simulink model "DCDCconverter"  (R2012b)
settings: Solver=ode3  StartTime=0.0  StopTime=inf  FixedStep=Tsample_simulink  RelTol=1e-3
PostLoadFcn:
  | , if any(exist('dsrtsu_mdlpostloadfcn', 'file') == [2, 3, 6]), try dsrtsu_mdlpostloadfcn('Execute', bdroot); catch fprintf('Error in PostLoadFcn (dsrtsu_mdlpostloadfcn) for model "%s":\n %s\n', bdroot, lasterr); end, end,
InitFcn:
  | load('../sim/me547_based_PI_controller_v3_saved_state.mat');
  | load('../sim/RuleBasedControlData_LeadAcid_48V_25C.mat');
undefined symbols (not defined in the file): BatVoltageLowerThresh, BatVoltageUpperThresh, C, DiscIntNeverNeededParam, Ea, fdesignblkfcn, gcbh, Icommand_Limit, Ireg_Integ_Limit, Kp_vc, MaxBatCurrent, MaxBatVoltage, MaxTemperature, MaxUCCurrent, MaxUCVoltage, Ra, RuleBasedControlHESSPowerValues, RuleBasedControlLUTValues, RuleBasedControlUCVoltageValues, TDelay_UltracapacitorRelay, Ts, Ts2, Tsample_simulink, UCVoltageLowerThresh, UCVoltageUpperThresh, Vbat, Vrail_rated
libraries: xpclib x35, rtilib1103 x8, dspsigops x5
(part 1 of 10)
settings Model: DSRTSU_INTERNAL_RTI_VER=430  DSRTSU_INTERNAL_RTI_TYPE=rti1103  DSRTSU_INTERNAL_RTIFPGA=20  TunableVars=Ea,Ra  TunableVarsStorageClass=Auto,Auto  TunableVarsTypeQualifier=,  BufferReuse=off  Creator=Renato  LastModifiedBy=Raghav
settings DataIOCC: SignalLoggingSaveFormat=ModelDataLogs
settings OptimizationCC: BlockReduction=off  OptimizeBlockIOStorage=off  BufferReuse=off  ExpressionFolding=off  ExpressionDepthLimit=128  LocalBlockOutputs=off
settings DebuggingCC: MultiTaskDSMMsg=warning  MultiTaskCondExecSysMsg=none  StrictBusMsg=None
settings HardwareCC: ProdIntDivRoundTo=Zero  ProdEndianess=BigEndian  ProdHWDeviceType=Generic->Custom  TargetIntDivRoundTo=Zero  TargetEndianess=BigEndian  TargetHWDeviceType=Generic->Custom
settings RTWCC: SystemTargetFile=rti1103.tlc  MakeCommand=make_rti  TemplateMakefile=rti1103.tmf  Description=dSPACE DS1103 Hardware Platform  ProcessScript=rti1103_make_rtw_hook  IncludeERTFirstTime=on
settings STFCustomTargetCC: CodeReplacementLibrary=ANSI_C  ParMdlRefBuildCompliant=on  GeneratePreprocessorConditionals=Disable all  SystemTargetFile=rti1103.tlc
settings GRTTargetCC: CompOptLevelCompliant=off  ConcurrentExecutionCompliant=off  CombineOutputUpdateFcns=off  MatFileLogging=off  GRTInterface=on  ExtModeMexFile=noextcomm

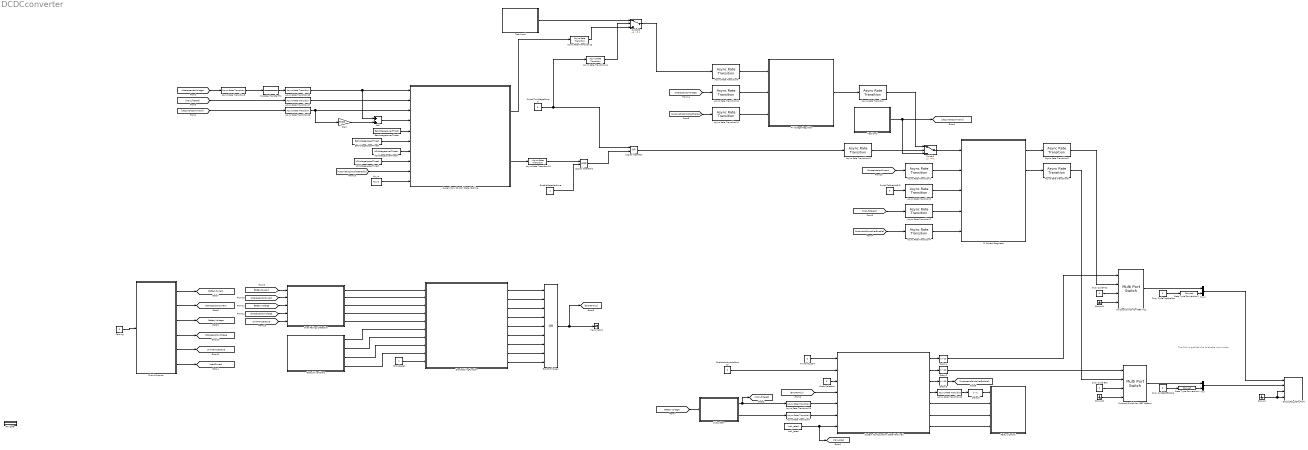
== system DCDCconverter ==
  note: The PWM is enabled whe its enable input is zero
  Add : Sum
  Async Rate Transition{,1..2,4..5,12} (6 alike) : xpclib/Asynchronous Event/Async Rate Transition  sample_time=Ts
  Async Rate Transition{8..11,13..14,16} (7 alike) : xpclib/Asynchronous Event/Async Rate Transition  sample_time=Ts2
  Async Rate Transition15 : xpclib/Asynchronous Event/Async Rate Transition  sample_time=2e-5
  Async Rate Transition17 : xpclib/Asynchronous Event/Async Rate Transition  sample_time=2e-5
  Async Rate Transition18 : xpclib/Asynchronous Event/Async Rate Transition  sample_time=2e-5
  Async Rate Transition19 : xpclib/Asynchronous Event/Async Rate Transition  sample_time=Tsample_simulink
  Async Rate Transition20 : xpclib/Asynchronous Event/Async Rate Transition  sample_time=TDelay_UltracapacitorRelay
  Async Rate Transition3 : xpclib/Asynchronous Event/Async Rate Transition  sample_time=0.00002
  Async Rate Transition6 : xpclib/Asynchronous Event/Async Rate Transition  sample_time=0.00002
  Async Rate Transition7 : xpclib/Asynchronous Event/Async Rate Transition  sample_time=Tsample_simulink
  BatVoltageLowerThresh : Constant  Value=BatVoltageLowerThresh
  BatVoltageUpperThresh : Constant  Value=BatVoltageUpperThresh
  Circuit Outputs : Subsystem
  DS1103SL_DSP_PWM : rtilib1103/DS1103 SLAVE DSP/DS1103SL_DSP_PWM  Parameters=[]  TDef=[]  BoardType=[]  PwmMode=[]  Frequency=[]  InitValue=[]  TermMode=[]  TermValue=[]  Polarity=[]  DialogFcn=[]  Reserved1=[]  Reserved2=[]  Reserved3=[]  Reserved4=[]  Revision=[]  UnitName=[]  UnitValues=[]  DSProperties=struct('RTI',struct('Version',uint32(2),'BlockType',struct('isSLSource',uint8(0),'isSLSink',uint8(1),'isHWSource',uint8(0),'isHWSink',uint8(1),'isSetup',uint8(0),'isInline',uint8(1),'isNonInline',uint8(0),'isInterrupt',uint8(0),'isChannelwise',uint8(0)),'IOBoardType','DS1103SLAVE','UnitType','PWM','Identifier','PWM','DialogType','ML','BlockSet','NONE','SlaveProcessor','F240'))  RTIBlockInterface=struct('InputPortsActive',[1 1 1 1],'InputPortsWidth',int32([2 2 2 2]),'InputPortsName',{{['PWM Channel 1'],['PWM Channel 2'],['PWM Channel 3'],['PWM Channel 4']}},'IWork',{{{'',uint32(4)}}},'DialogFcn','rti1103slavepwmgui','InitLevel',1,'BlockDisplay',{{'','auto'}},'IconTransparency','on','MultiSFcn',4,'BlockName',struct('Token',{{'DS1103SL_DSP_PWM'}}))  RTIBlockParameters=struct('PWMSymmetryMode',{{1,'OFF',[]}},'PWMFrequency',{{'5000','OFF',[]}},'PWMPolarityMode',{{[1 1 1 1 1],'OFF',[]}},'ChannelNo',{{[1 2 3 4],'OFF',[]}},'SuspendModeInit',{{[1 1 1 1 1],'OFF',[]}},'TTLModeInit',{{[2 2 2 2 2],'OFF',[]}},'DutyCycleInitValueCh1',{{'0.5','OFF',[]}},'DutyCycleInitValueCh2',{{'0.5','OFF',[]}},'DutyCycleInitValueCh3',{{'0.5','OFF',[]}},'DutyCycleInitValueCh4',{{'0.5','OFF',[]}},'DutyCycleInitValueCh5',{{'0.5','OFF',[]}},'EnablePWMStop',{{[1 1 1 1 0],'OFF',[]}},'SuspendModeTerm',{{[1 1 1 1 1],'OFF',[]}},'TTLModeTerm',{{[2 2 2 2 2],'OFF',[]}},'DutyCycleTermValueCh1',{{'0.5','OFF',[]}},'DutyCycleTermValueCh2',{{'0.5','OFF',[]}},'DutyCycleTermValueCh3',{{'0.5','OFF',[]}},'DutyCycleTermValueCh4',{{'0.5','OFF',[]}},'DutyCycleTermValueCh5',{{'0.5','OFF',[]}},'TLCFileName',{{'rti1103pwm','OFF',[]}})  RTISFcnParameters=struct('PWMSymmetryMode','double','PWMFrequency','double','PWMPolarityMode','double','ChannelNo','double','SuspendModeInit','double','TTLModeInit','double','DutyCycleInitValueCh1','double','DutyCycleInitValueCh2','double','DutyCycleInitValueCh3','double','DutyCycleInitValueCh4','double','EnablePWMStop','double','SuspendModeTerm','double','TTLModeTerm','double','DutyCycleTermValueCh1','double','DutyCycleTermValueCh2','double','DutyCycleTermValueCh3','double','DutyCycleTermValueCh4','double','TLCFileName','char')  RTIBlockParaDefault=struct('PWMSymmetryMode',1,'PWMFrequency',100,'PWMPolarityMode',[1 1 1 1 1],'ChannelNo',[1 2 3 4],'SuspendModeInit',[1 1 1 1 1],'TTLModeInit',[2 2 2 2 2],'DutyCycleInitValueCh1',0.5,'DutyCycleInitValueCh2',0.5,'DutyCycleInitValueCh3',0.5,'DutyCycleInitValueCh4',0.5,'DutyCycleInitValueCh5',0.5,'EnablePWMStop',[1 1 1 1 0],'SuspendModeTerm',[1 1 1 1 1],'TTLModeTerm',[2 2 2 2 2],'DutyCycleTermValueCh1',0.5,'DutyCycleTermValueCh2',0.5,'DutyCycleTermValueCh3',0.5,'DutyCycleTermValueCh4',0.5,'DutyCycleTermValueCh5',0.5,'TLCFileName','rti1103pwm')
  Data Type Conversion1 : DataTypeConversion
  Data Type Conversion2 : DataTypeConversion
  Delay1 : Delay  DelayLength=10  SampleTime=Tsample_simulink
  Delay2 : Delay  DelayLength=10  SampleTime=Tsample_simulink
  Delay3 : Delay  DelayLength=10  SampleTime=Tsample_simulink
  Delay5 : Delay  DelayLength=1  SampleTime=TDelay_UltracapacitorRelay
  Discrete Transfer Fcn : DiscreteTransferFcn  Numerator=[1 1 1 1]  Denominator=[4 0 0 0]  SampleTime=Ts2
  Duty Cycle Bot : Constant  Value=0
  Duty CycleBotEnable : Constant  Value=0
  Duty CycleTop : Constant  Value=0
  Duty CycleTopEnable : Constant  Value=0
  EnableAutomaticControl : Constant  Value=0
  EnableStateMachine : Constant  SampleTime=-1
  ErrorForTripNew : Logic  Operator=OR  Inputs=9  AllPortsSameDT=off  OutDataTypeStr=boolean
  ErrorLatchingFunction : MATLAB Function  TreatAsAtomicUnit=on
  Error_Reset : Constant
  Gain : Gain  Gain=Ts2/C
  Gate Driver Errors : Subsystem
  Ground : Ground
  Ground1 : Ground
  Ground2 : Ground
  Kp_vc : Constant  Value=Kp_vc  SampleTime=-1
  Logical Operator : Logic  Operator=OR  AllPortsSameDT=off  OutDataTypeStr=boolean
  Logical Operator1 : Logic  AllPortsSameDT=off  OutDataTypeStr=boolean
  Mode Selection : Constant  Value=0
  Multiport Switch for IGBT Bottom : MultiPortSwitch  Inputs=2  DataPortForDefault=Additional data port  DiagnosticForDefault=None
  Multiport Switch for IGBT Top : MultiPortSwitch  Inputs=2  DataPortForDefault=Additional data port  DiagnosticForDefault=None
  Mux : Mux  Inputs=2
  Mux1 : Mux  Inputs=2
  Over Ratings Detection : Subsystem
  PI Current Regulator : Subsystem
  PI Voltage Regulator : Subsystem
  RTI Data : Subsystem  Tag=struct('RTIDataServer',struct('RTIDataServerVs','2','RTIModelDescription','struct(''main'',''DCDCconverter'',''sub'','''',''isMp'',0)'))  LoadFcn="if exist('rtidc'), try,  rtidc('DataHostBlockClbLoad', gcbh); catch, disp(['Warning: ''LoadFcn'' for RTI Data block failed: ' lasterr]); end, end,"  mask(RTI_DATA_HOST){}
      mask help:
      | RTI Data Block.
      | This block is used by RTI to store internal model-dependent data.
      | Please keep this block on the root level of the model. Deleting this block will result in data loss.
      |
      | NEVER DELETE OR COPY THIS BLOCK!
      settings: CopyFcn="if exist('rtidc'), try,  rtidc('DataHostBlockClbCopy', gcbh); catch, disp(['Warning: ''CopyFcn'' for RTI Data block failed: ' lasterr]); end, end,"  DeleteFcn="if exist('rtidc'), try,  rtidc('DataHostBlockClbDelete', gcbh); catch, disp(['Warning: ''DeleteFcn'' for RTI Data block failed: ' lasterr]); end, end,"  ModelCloseFcn="if exist('rtidc'), try,  rtidc('DataHostBlockClbModelClose', gcbh); catch, disp(['Warning: ''ModelCloseFcn'' for RTI Data block failed: ' lasterr]); end, end,"  PreSaveFcn="if exist('rtidc'), try,  rtidc('DataHostBlockClbPreSave', gcbh); catch, disp(['Warning: ''PreSaveFcn'' for RTI Data block failed: ' lasterr]); end, end,"  PostSaveFcn="if exist('rtidc'), try,  rtidc('DataHostBlockClbPostSave', gcbh); catch, disp(['Warning: ''PostSaveFcn'' for RTI Data block failed: ' lasterr]); end, end,"  NameChangeFcn="if exist('rtidc'), try,  rtidc('DataHostBlockClbNameChange', gcbh); catch, disp(['Warning: ''NameChangeFcn'' for RTI Data block failed: ' lasterr]); end, end,"
      mask Help:
      | RTI Data Block.
      | This block is used by RTI to store internal model-dependent data.
      | Please keep this block on the root level of the model. Deleting this block will result in data loss.
      | 
      | NEVER DELETE OR COPY THIS BLOCK!
      mask Display:
      | text(0.5, 0.5, 'RTI Data', 'HorizontalAlignment', 'center');
      | plot([1 0]);
  Relays Control : Subsystem
  Subsystem : Subsystem
  Supervisory Control State Machine : Stateflow chart  TreatAsAtomicUnit=on
  Switch2 : Switch  Threshold=1  OutDataTypeStr=Inherit: Inherit via back propagation  SampleTime=Ts
  Switch5 : Switch  Threshold=1  OutDataTypeStr=Inherit: Inherit via back propagation  SampleTime=Ts2
  SwitchToEnableDID : Constant  Value=0
  SwitchToVoltageControl : Constant  Value=0  SampleTime=-1
  System Configuration State Machine1 : Stateflow chart  TreatAsAtomicUnit=on
  Terminator1 : Terminator
  Test Icmd : Subsystem
  Test Vcmd : Subsystem
  TurnOnSystem : Constant  Value=0
  UCVoltageLowerThresh : Constant  Value=UCVoltageLowerThresh
  UCVoltageUpperThresh : Constant  Value=UCVoltageUpperThresh
  Vrail_rated : Constant  Value=Vrail_rated
  Zeroing : Constant  Value=0
  tag scope: BatteryCurrent=global, BatteryVoltage=global, LoadCurrent=global, SinkTemperature=global, UltracapacitorCurrent=global, UltracapacitorVoltage=global, Vrail_rated=global
  wires:
  Data Type Conversion1/1 -> Mux/2
  Over Ratings Detection/5(Temperature Alert) -> ErrorLatchingFunction/5(TempAlert)
  Over Ratings Detection/4(Ultracapacitor Voltage Alert) -> ErrorLatchingFunction/4(UCVoltageAlert)
  Over Ratings Detection/3(Battery Voltage Alert) -> ErrorLatchingFunction/3(BatVoltageAlert)
  Over Ratings Detection/2(Ultra Capacitor Current Alert) -> ErrorLatchingFunction/2(UCCurrentAlert)
  Over Ratings Detection/1(Battery Current Alert) -> ErrorLatchingFunction/1(BatCurrentAlert)
  Mux/1 -> DS1103SL_DSP_PWM/2
  Gate Driver Errors/1(Error HB1) -> ErrorLatchingFunction/6(ErrorHB1)
  Gate Driver Errors/2(Error HB2) -> ErrorLatchingFunction/7(ErrorHB2)
  Gate Driver Errors/3(Error HB3) -> ErrorLatchingFunction/8(ErrorHB3)
  Gate Driver Errors/4(Over Temperature) -> ErrorLatchingFunction/9(OverTemp)
  Duty CycleTop/1 -> Multiport Switch for IGBT Top/3
  Data Type Conversion2/1 -> Mux1/2
  Mux1/1 -> DS1103SL_DSP_PWM/1
  Ground/1 -> DS1103SL_DSP_PWM/3, DS1103SL_DSP_PWM/4
  Zeroing/1 -> Circuit Outputs/1(Zeroing)
  Multiport Switch for IGBT Top/1 -> Mux1/1
  Multiport Switch for IGBT Bottom/1 -> Mux/1
  PI Current Regulator/1(Duty Cycle Command Top) -> Async Rate Transition3/1
  Duty Cycle Bot/1 -> Multiport Switch for IGBT Bottom/3
  EnableAutomaticControl/1 -> System Configuration State Machine1/2(EnableAutomaticControl)
  Async Rate Transition1/1 -> PI Current Regulator/2(Avg Current Measurement)
  Async Rate Transition2/1 -> PI Current Regulator/4(DC Bus Voltage Measurement)
  SwitchToEnableDID/1 -> Async Rate Transition5/1
  Async Rate Transition4/1 -> PI Current Regulator/5(Enable PI Controller)
  Async Rate Transition5/1 -> PI Current Regulator/3(Enable DID)
  PI Current Regulator/2(Duty Cycle Command Bottom) -> Async Rate Transition6/1
  Duty CycleTopEnable/1 -> Data Type Conversion2/1
  Duty CycleBotEnable/1 -> Data Type Conversion1/1
  Async Rate Transition3/1 -> Multiport Switch for IGBT Top/2
  Async Rate Transition6/1 -> Multiport Switch for IGBT Bottom/2
  Async Rate Transition9/1 -> PI Voltage Regulator/1(UC Voltage Command)
  Async Rate Transition10/1 -> PI Voltage Regulator/2(UC Voltage Measurement)
  Async Rate Transition11/1 -> PI Voltage Regulator/3(Enable PI Controller)
  Test Icmd/1(Current Command) -> [UCCurrentCommand], Switch2/3
  PI Voltage Regulator/1(Avg Current Command) -> Async Rate Transition/1
  Switch2/1 -> PI Current Regulator/1(Avg Current Command)
  Async Rate Transition/1 -> Switch2/1
  BatVoltageLowerThresh/1 -> Supervisory Control State Machine/5(BatVoltageLowerThresh)
  BatVoltageUpperThresh/1 -> Supervisory Control State Machine/6(BatVoltageUpperThresh)
  UCVoltageLowerThresh/1 -> Supervisory Control State Machine/7(UCVoltageLowerThresh)
  UCVoltageUpperThresh/1 -> Supervisory Control State Machine/8(UCVoltageUpperThresh)
  Supervisory Control State Machine/2(EnableVoltageCommand) -> Async Rate Transition16/1
  EnableStateMachine/1 -> Logical Operator1/2
  Test Vcmd/1(Voltage Command) -> Switch5/1
  Switch5/1 -> Async Rate Transition9/1
  [UltracapacitorVoltage] -> Async Rate Transition8/1
  Gain/1 -> Add/2
  Logical Operator/1 -> Async Rate Transition12/1
  Logical Operator1/1 -> Logical Operator/2
  Async Rate Transition12/1 -> Switch2/2
  Supervisory Control State Machine/1(VoltageCommand) -> Async Rate Transition13/1
  SwitchToVoltageControl/1 -> Async Rate Transition14/1, Logical Operator/1
  Discrete Transfer Fcn/1 -> Async Rate Transition15/1
  [Vrail_filtered] -> Async Rate Transition17/1
  [UCCurrentCommand] -> Async Rate Transition18/1
  Async Rate Transition13/1 -> Switch5/3
  Async Rate Transition14/1 -> Switch5/2
  Async Rate Transition15/1 -> Supervisory Control State Machine/1(Average_UCVoltage), Add/1
  Async Rate Transition17/1 -> Supervisory Control State Machine/2(Average_BatVoltage)
  Async Rate Transition18/1 -> Supervisory Control State Machine/3(UCCurrentCommand), Gain/1
  Add/1 -> Supervisory Control State Machine/4(UCVoltage_next_predicted)
  Ground1/1 -> Multiport Switch for IGBT Top/4
  Ground2/1 -> Multiport Switch for IGBT Bottom/4
  Delay2/1 -> Multiport Switch for IGBT Bottom/1
  Subsystem/1(Vrail_filtered) -> Async Rate Transition19/1, [Vrail_filtered]
  Subsystem/2(dVrail_dT_filtered) -> Async Rate Transition7/1
  [Vrail_filtered] -> Async Rate Transition2/1
  Async Rate Transition19/1 -> System Configuration State Machine1/5(Vrail)
  Async Rate Transition7/1 -> System Configuration State Machine1/6(dVrail_dT)
  Vrail_rated/1 -> [Vrail_rated], System Configuration State Machine1/7(Vrail_rated)
  [ErrorForTrip] -> System Configuration State Machine1/4(Error)
  Mode Selection/1 -> System Configuration State Machine1/3(ManualControlBuckMode)
  System Configuration State Machine1/4(UltracapacitorRelay) -> Async Rate Transition20/1
  System Configuration State Machine1/5(ChargingRelay) -> Relays Control/2(Charging Relay)
  System Configuration State Machine1/6(DischargingRelay) -> Relays Control/3(Discharging Relay)
  System Configuration State Machine1/7(BatteryRelay) -> Relays Control/4(Battery Relay)
  Delay3/1 -> [AutomaticControllerEnable]
  Circuit Outputs/1(Battery Current) -> [BatteryCurrent]
  Circuit Outputs/2(UltraCapacitor Current) -> [UltracapacitorCurrent]
  Circuit Outputs/3(Battery Voltage) -> [BatteryVoltage]
  Circuit Outputs/4(UltraCapacitor Voltage) -> [UltracapacitorVoltage]
  Circuit Outputs/5(Sink Temperature) -> [SinkTemperature]
  [BatteryVoltage] -> Subsystem/1(Vrail)
  TurnOnSystem/1 -> System Configuration State Machine1/1(TurnOnSystem)
  [AutomaticControllerEnable] -> Async Rate Transition4/1
  [AutomaticControllerEnable] -> Async Rate Transition11/1
  Delay1/1 -> Multiport Switch for IGBT Top/1
  System Configuration State Machine1/2(IGBT_Bot_State) -> Delay2/1
  System Configuration State Machine1/3(AutomaticController) -> Delay3/1
  System Configuration State Machine1/1(IGBT_Top_State) -> Delay1/1
  [BatteryCurrent] -> Over Ratings Detection/1(Battery Current)
  [UltracapacitorCurrent] -> Over Ratings Detection/2(Ultra Capacitor Current)
  [BatteryVoltage] -> Over Ratings Detection/3(Battery Voltage)
  [UltracapacitorVoltage] -> Over Ratings Detection/4(Ultra Capacitor Voltage)
  [SinkTemperature] -> Over Ratings Detection/5(Temperature)
  [UltracapacitorVoltage] -> Async Rate Transition10/1
  [UltracapacitorCurrent] -> Async Rate Transition1/1
  [AutomaticControllerEnable] -> Supervisory Control State Machine/9(AutomaticControllerEnable)
  Kp_vc/1 -> Supervisory Control State Machine/10(Kp_vc)
  ErrorLatchingFunction/3(LBatVoltageAlert) -> ErrorForTripNew/3
  ErrorLatchingFunction/2(LUCCurrentAlert) -> ErrorForTripNew/2
  ErrorLatchingFunction/4(LUCVoltageAlert) -> ErrorForTripNew/4
  ErrorLatchingFunction/7(LErrorHB2) -> ErrorForTripNew/7
  ErrorLatchingFunction/5(LTempAlert) -> ErrorForTripNew/5
  ErrorLatchingFunction/8(LErrorHB3) -> ErrorForTripNew/8
  ErrorLatchingFunction/6(LErrorHB1) -> ErrorForTripNew/6
  ErrorLatchingFunction/9(LOverTemp) -> ErrorForTripNew/9
  ErrorLatchingFunction/1(LBatCurrentAlert) -> ErrorForTripNew/1
  ErrorForTripNew/1 -> [ErrorForTrip], Terminator1/1
  Error_Reset/1 -> ErrorLatchingFunction/10(Error_Reset)
  Async Rate Transition8/1 -> Discrete Transfer Fcn/1
  Circuit Outputs/6(Load Current) -> [LoadCurrent]
  Async Rate Transition16/1 -> Logical Operator1/1
  Delay5/1 -> Relays Control/1(UltraCapacitor Relay)
  Async Rate Transition20/1 -> Delay5/1

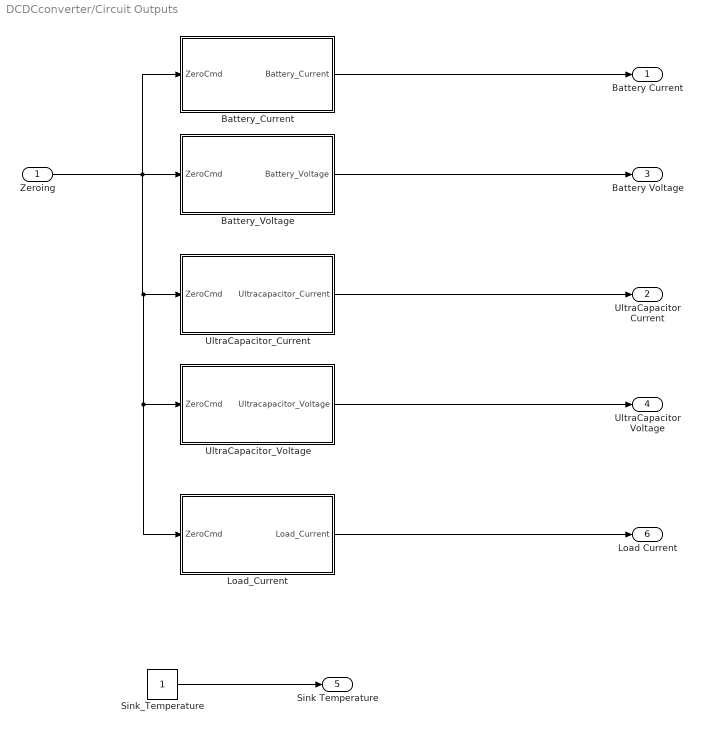
== system DCDCconverter/Circuit Outputs ==
  Zeroing : Inport
  Battery_Current : Subsystem
  Battery_Voltage : Subsystem
  Load_Current : Subsystem
  Sink_Temperature : Constant
  UltraCapacitor_Current : Subsystem
  UltraCapacitor_Voltage : Subsystem
  Battery Current : Outport
  UltraCapacitor Current : Outport  Port=2
  Battery Voltage : Outport  Port=3
  UltraCapacitor Voltage : Outport  Port=4
  Sink Temperature : Outport  Port=5
  Load Current : Outport  Port=6
  wires:
  Battery_Voltage/1(Battery_Voltage) -> Battery Voltage/1
  Battery_Current/1(Battery_Current) -> Battery Current/1
  Sink_Temperature/1 -> Sink Temperature/1
  Zeroing/1 -> Load_Current/1(ZeroCmd), UltraCapacitor_Voltage/1(ZeroCmd), UltraCapacitor_Current/1(ZeroCmd), Battery_Voltage/1(ZeroCmd), Battery_Current/1(ZeroCmd)
  UltraCapacitor_Voltage/1(Ultracapacitor_Voltage) -> UltraCapacitor Voltage/1
  UltraCapacitor_Current/1(Ultracapacitor_Current) -> UltraCapacitor Current/1
  Load_Current/1(Load_Current) -> Load Current/1

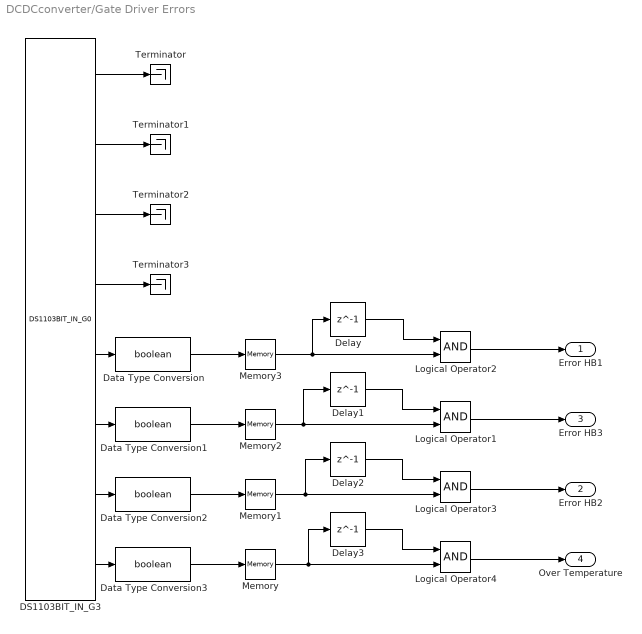
== system DCDCconverter/Gate Driver Errors ==
  DS1103BIT_IN_G3 : rtilib1103/DS1103 MASTER PPC/DS1103BIT_IN_G0  GroupNo=3  Reserved1=[]  Reserved2=[]  Reserved3=[]  Reserved4=[]  DialogFcn=gui1103bit_inx  UnitName={ 'DS1103BIT_IN_G'}  UnitValues={ 3 }  DSProperties=struct('RTI',struct('Version',uint32(1),'BlockType',struct('isSLSource',uint8(1),'isSLSink',uint8(0),'isHWSource',uint8(1),'isHWSink',uint8(0),'isSetup',uint8(0),'isInline',uint8(1),'isNonInline',uint8(0),'isInterrupt',uint8(0),'isChannelwise',uint8(0)),'IOBoardType','DS1103MASTER','UnitType','BIT','Identifier','BITIN','DialogType','ML','BlockSet','NONE','SlaveProcessor','NONE'))
  Data Type Conversion{,1..3} (4 alike) : DataTypeConversion  OutDataTypeStr=boolean
  Delay{,1..3} (4 alike) : Delay  DelayLength=1
  Logical Operator{1..4} (4 alike) : Logic  AllPortsSameDT=off  OutDataTypeStr=boolean
  Memory{,1..3} (4 alike) : Memory  InheritSampleTime=on
  Terminator{,1..3} (4 alike) : Terminator
  Error HB1 : Outport
  Error HB2 : Outport  Port=2
  Error HB3 : Outport  Port=3
  Over Temperature : Outport  Port=4
  wires:
  DS1103BIT_IN_G3/1 -> Terminator/1
  DS1103BIT_IN_G3/4 -> Terminator3/1
  DS1103BIT_IN_G3/2 -> Terminator1/1
  DS1103BIT_IN_G3/3 -> Terminator2/1
  DS1103BIT_IN_G3/8 -> Data Type Conversion3/1
  DS1103BIT_IN_G3/6 -> Data Type Conversion1/1
  DS1103BIT_IN_G3/7 -> Data Type Conversion2/1
  DS1103BIT_IN_G3/5 -> Data Type Conversion/1
  Data Type Conversion3/1 -> Memory/1
  Data Type Conversion2/1 -> Memory1/1
  Data Type Conversion1/1 -> Memory2/1
  Data Type Conversion/1 -> Memory3/1
  Memory3/1 -> Delay/1, Logical Operator2/2
  Logical Operator2/1 -> Error HB1/1
  Delay/1 -> Logical Operator2/1
  Memory2/1 -> Delay1/1, Logical Operator1/2
  Logical Operator1/1 -> Error HB3/1
  Delay1/1 -> Logical Operator1/1
  Logical Operator3/1 -> Error HB2/1
  Memory1/1 -> Delay2/1, Logical Operator3/2
  Delay2/1 -> Logical Operator3/1
  Logical Operator4/1 -> Over Temperature/1
  Memory/1 -> Logical Operator4/2, Delay3/1
  Delay3/1 -> Logical Operator4/1

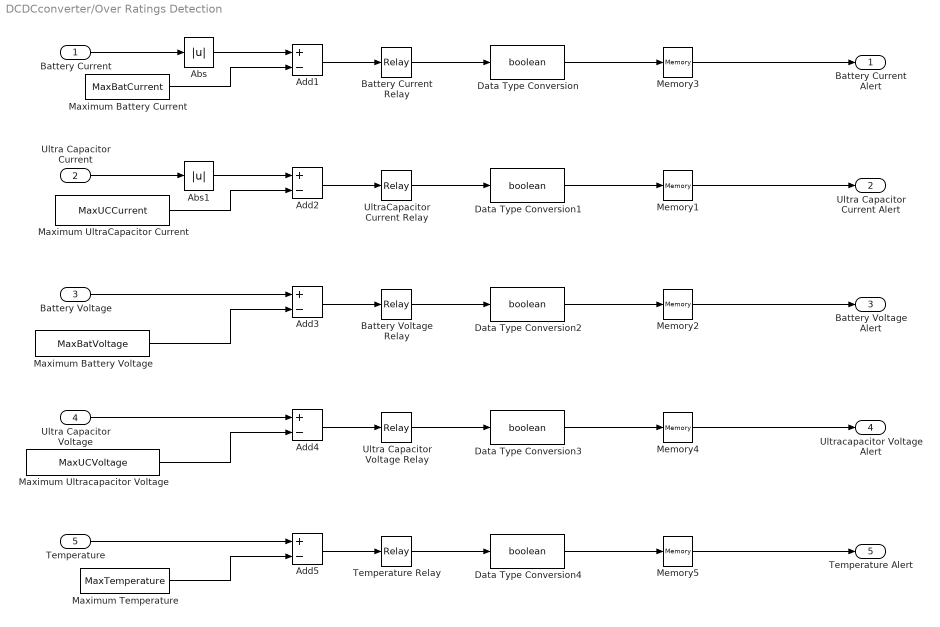
== system DCDCconverter/Over Ratings Detection ==
  Battery Current : Inport
  Ultra Capacitor Current : Inport  Port=2
  Battery Voltage : Inport  Port=3
  Ultra Capacitor Voltage : Inport  Port=4
  Temperature : Inport  Port=5
  Abs : Abs
  Abs1 : Abs
  Add{1..5} (5 alike) : Sum  Inputs=+-
  Battery Current Relay : Relay  OnSwitchValue=0  OffSwitchValue=0
  Battery Voltage Relay : Relay  OnSwitchValue=0  OffSwitchValue=0
  Data Type Conversion{,1..4} (5 alike) : DataTypeConversion  OutDataTypeStr=boolean
  Maximum Battery Current : Constant  Value=MaxBatCurrent
  Maximum Battery Voltage : Constant  Value=MaxBatVoltage
  Maximum Temperature : Constant  Value=MaxTemperature
  Maximum UltraCapacitor Current : Constant  Value=MaxUCCurrent
  Maximum Ultracapacitor Voltage : Constant  Value=MaxUCVoltage
  Memory{1..5} (5 alike) : Memory  InheritSampleTime=on
  Temperature Relay : Relay  OnSwitchValue=0  OffSwitchValue=0
  Ultra Capacitor Voltage Relay : Relay  OnSwitchValue=0  OffSwitchValue=0
  UltraCapacitor Current Relay : Relay  OnSwitchValue=0  OffSwitchValue=0
  Battery Current Alert : Outport
  Ultra Capacitor Current Alert : Outport  Port=2
  Battery Voltage Alert : Outport  Port=3
  Ultracapacitor Voltage Alert : Outport  Port=4
  Temperature Alert : Outport  Port=5
  wires:
  Add3/1 -> Battery Voltage Relay/1
  Maximum Battery Voltage/1 -> Add3/2
  Battery Voltage/1 -> Add3/1
  Add4/1 -> Ultra Capacitor Voltage Relay/1
  Maximum Ultracapacitor Voltage/1 -> Add4/2
  Ultra Capacitor Voltage/1 -> Add4/1
  Add2/1 -> UltraCapacitor Current Relay/1
  Maximum UltraCapacitor Current/1 -> Add2/2
  Ultra Capacitor Current/1 -> Abs1/1
  Add5/1 -> Temperature Relay/1
  Maximum Temperature/1 -> Add5/2
  Temperature/1 -> Add5/1
  Add1/1 -> Battery Current Relay/1
  Maximum Battery Current/1 -> Add1/2
  Battery Current/1 -> Abs/1
  Battery Current Relay/1 -> Data Type Conversion/1
  UltraCapacitor Current Relay/1 -> Data Type Conversion1/1
  Battery Voltage Relay/1 -> Data Type Conversion2/1
  Ultra Capacitor Voltage Relay/1 -> Data Type Conversion3/1
  Temperature Relay/1 -> Data Type Conversion4/1
  Data Type Conversion/1 -> Memory3/1
  Data Type Conversion1/1 -> Memory1/1
  Data Type Conversion2/1 -> Memory2/1
  Data Type Conversion3/1 -> Memory4/1
  Data Type Conversion4/1 -> Memory5/1
  Memory3/1 -> Battery Current Alert/1
  Memory1/1 -> Ultra Capacitor Current Alert/1
  Memory2/1 -> Battery Voltage Alert/1
  Memory4/1 -> Ultracapacitor Voltage Alert/1
  Memory5/1 -> Temperature Alert/1
  Abs/1 -> Add1/1
  Abs1/1 -> Add2/1

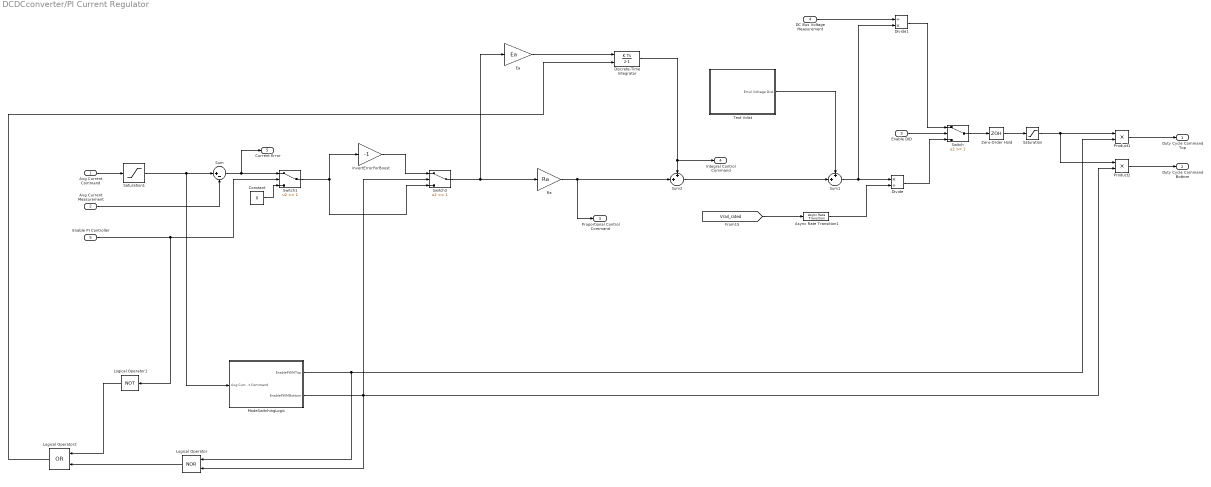
== system DCDCconverter/PI Current Regulator ==
  Avg Current Command : Inport
  Avg Current Measurement : Inport  Port=2
  Enable DID : Inport  Port=3
  DC Bus Voltage Measurement : Inport  Port=4
  Enable PI Controller : Inport  Port=5
  Async Rate Transition1 : xpclib/Asynchronous Event/Async Rate Transition  sample_time=Ts
  Constant : Constant  Value=0  SampleTime=Ts
  Discrete-Time Integrator : DiscreteIntegrator  ExternalReset=either  SampleTime=Ts  LimitOutput=on  UpperSaturationLimit=Ireg_Integ_Limit  LowerSaturationLimit=-Ireg_Integ_Limit  ICPrevOutput=DiscIntNeverNeededParam  ICPrevScaledInput=DiscIntNeverNeededParam
  Divide : Product  Inputs=*/
  Divide1 : Product  Inputs=/*
  Ea : Gain  Gain=Ea  SampleTime=Ts
  InvertErrorForBoost : Gain  Gain=-1  SampleTime=Ts
  Logical Operator : Logic  Operator=NOR  AllPortsSameDT=off  OutDataTypeStr=boolean
  Logical Operator1 : Logic  Operator=NOT  AllPortsSameDT=off  OutDataTypeStr=boolean
  Logical Operator2 : Logic  Operator=OR  AllPortsSameDT=off  OutDataTypeStr=boolean
  ModeSwitchingLogic : Subsystem
  Product1 : Product  RndMeth=Zero
  Product2 : Product  RndMeth=Zero
  Ra : Gain  Gain=Ra  SampleTime=Ts
  Saturation : Saturate  UpperLimit=1  LowerLimit=0
  Saturation1 : Saturate  UpperLimit=Icommand_Limit  LowerLimit=-Icommand_Limit
  Sum : Sum  Inputs=|+-
  Sum1 : Sum  Inputs=++|
  Sum2 : Sum  Inputs=++|
  Switch : Switch  Threshold=1
  Switch1 : Switch  Threshold=1
  Switch3 : Switch  Threshold=1
  Test Vdist : Subsystem
  Zero-Order Hold : ZeroOrderHold  SampleTime=Ts
  Duty Cycle Command Top : Outport
  Duty Cycle Command Bottom : Outport  Port=2
  Proportional Control Command : Outport  Port=3
  Integral Control Command : Outport  Port=4
  Current Error : Outport  Port=5
  wires:
  Divide/1 -> Switch/3
  Ea/1 -> Discrete-Time Integrator/1
  Zero-Order Hold/1 -> Saturation/1
  Ra/1 -> Proportional Control Command/1, Sum2/2
  Discrete-Time Integrator/1 -> Sum2/1, Integral Control Command/1
  Switch/1 -> Zero-Order Hold/1
  Enable DID/1 -> Switch/2
  DC Bus Voltage Measurement/1 -> Divide1/1
  Divide1/1 -> Switch/1
  Sum/1 -> Current Error/1, Switch1/1
  Constant/1 -> Switch1/3
  Avg Current Command/1 -> Saturation1/1
  Avg Current Measurement/1 -> Sum/2
  Enable PI Controller/1 -> Logical Operator1/1, Switch1/2
  Saturation/1 -> Product2/1, Product1/1
  ModeSwitchingLogic/1(EnablePWMTop) -> Product1/2, Logical Operator/1
  ModeSwitchingLogic/2(EnablePWMBottom) -> Logical Operator/2, Product2/2, Switch3/2
  Sum2/1 -> Sum1/2
  Sum1/1 -> Divide1/2, Divide/1
  Test Vdist/1(Emul Voltage Dist) -> Sum1/1
  Logical Operator2/1 -> Discrete-Time Integrator/2
  Switch1/1 -> Switch3/3, InvertErrorForBoost/1
  InvertErrorForBoost/1 -> Switch3/1
  Switch3/1 -> Ea/1, Ra/1
  Saturation1/1 -> ModeSwitchingLogic/1(Avg Current Command), Sum/1
  Logical Operator1/1 -> Logical Operator2/1
  Logical Operator/1 -> Logical Operator2/2
  Product1/1 -> Duty Cycle Command Top/1
  Product2/1 -> Duty Cycle Command Bottom/1
  [Vrail_rated] -> Async Rate Transition1/1
  Async Rate Transition1/1 -> Divide/2

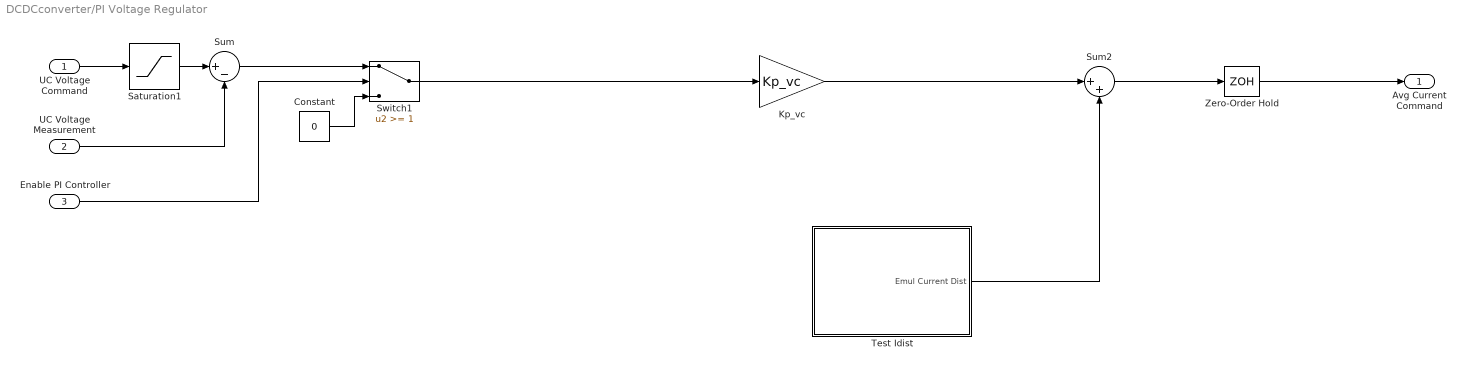
== system DCDCconverter/PI Voltage Regulator ==
  UC Voltage Command : Inport
  UC Voltage Measurement : Inport  Port=2
  Enable PI Controller : Inport  Port=3
  Constant : Constant  Value=0  SampleTime=Ts2
  Kp_vc : Gain  Gain=Kp_vc  SampleTime=Ts2
  Saturation1 : Saturate  UpperLimit=Vbat-1  LowerLimit=0
  Sum : Sum  Inputs=|+-
  Sum2 : Sum  Inputs=|++
  Switch1 : Switch  Threshold=1
  Test Idist : Subsystem
  Zero-Order Hold : ZeroOrderHold  SampleTime=Ts2
  Avg Current Command : Outport
  wires:
  Switch1/1 -> Kp_vc/1
  Sum/1 -> Switch1/1
  Constant/1 -> Switch1/3
  UC Voltage Command/1 -> Saturation1/1
  UC Voltage Measurement/1 -> Sum/2
  Enable PI Controller/1 -> Switch1/2
  Zero-Order Hold/1 -> Avg Current Command/1
  Saturation1/1 -> Sum/1
  Sum2/1 -> Zero-Order Hold/1
  Kp_vc/1 -> Sum2/1
  Test Idist/1(Emul Current Dist) -> Sum2/2

== system DCDCconverter/RTI Data ==
  RTI Data Store : Subsystem  Tag="struct('public',struct('sub',struct('name',{{'DCDCconverter'}},'data',{{struct('TH',struct('thTaskInfo',struct('taskType',{'TIMER','HWINT','TMRINT','SWINT','GLINT'},'tasksNumOf',{4,0,0,0,0},'srcIds',{{'TIMERA','TIMERA2','TIMERA3','TIMERA4'},{},{},{},{}},'taskNames',{{['Timer Task 1'],['Timer Task 2'],['Timer Task 3'],['Timer Task 4']},{},{},{},{}})),'th_tc',struct('dataType',{'TASK','TASK','TASK','TASK'},'taskGroupId',{'','','',''},'taskGroupList',{{},{},{},{}},'taskSchedulingPolicy',{'FCFS','FCFS','FCFS','FCFS'},'taskType',{'TIMER','TIMER','TIMER','TIMER'},'blkh',{-1,-1,-1,-1},'srcId',{'TIMERA','TIMERA2','TIMERA3','TIMERA4'},'srcSgnName',{['Timer A interrupt'],['Timer Task 1'],['Timer Task 1'],['Timer Task 1']},'srcCpuName',{'','','',''},'taskName',{['Timer Task 1  [2e-05] s'],['Timer Task 2  [0.0002] s'],['Timer Task 3  [0.05] s'],['Timer Task 4  [0.5] s']},'taskNameDisplayExt',{'','','',''},'smplTime',{2e-05,0.0002,0.05,0.5},'smplTimeOffs',{0,0,0,0},'hasFixedPriority',{0,0,0,0},'priority',{1,2,3,4},'hasFixedOvc',{0,0,0,0},'ovcType',{1,1,1,1},'ovcMax',{1,1,1,1}),'tc_th',struct('dataType',{'TASK','TASK','TASK','TASK'},'taskGroupId',{'','','',''},'taskGroupList',{{},{},{},{}},'taskSchedulingPolicy',{'FCFS','FCFS','FCFS','FCFS'},'taskType',{'TIMER','TIMER','TIMER','TIMER'},'blkh',{-1,-1,-1,-1},'srcId',{'TIMERA','TIMERA2','TIMERA3','TIMERA4'},'srcSgnName',{['Timer A interrupt'],['Timer Task 1'],['Timer Task 1'],['Timer Task 1']},'srcCpuName',{'','','',''},'taskName',{['Timer Task 1  [2e-05] s'],['Timer Task 2  [0.0002] s'],['Timer Task 3  [0.05] s'],['Timer Task 4  [0.5] s']},'taskNameDisplayExt',{'','','',''},'smplTime',{2e-05,0.0002,0.05,0.5},'smplTimeOffs',{0,0,0,0},'hasFixedPriority',{0,0,0,0},'priority',{1,2,3,4},'hasFixedOvc',{0,0,0,0},'ovcType',{1,1,1,1},'ovcMax',{1,1,1,1}))}})),'private',struct('version',struct('dsVer',uint32(2)),'access',struct('modified',['07-Aug-2015 20:22:16'],'type','Model','isPerm',1)))"  mask(RTI_DATA_STORE){}
      mask help:
      | RTI Data Store Block. This block is used by RTI to store internal model dependent data. Deleting this block will result in data loss.
      |
      | NEVER DELETE, COPY, OR MODIFY THIS BLOCK!
      mask Help:
      | RTI Data Store Block. This block is used by RTI to store internal model dependent data. Deleting this block will result in data loss.
      | 
      | NEVER DELETE, COPY, OR MODIFY THIS BLOCK!
      mask Display: text(0.5, 0.5, ' ', 'HorizontalAlignment', 'center');

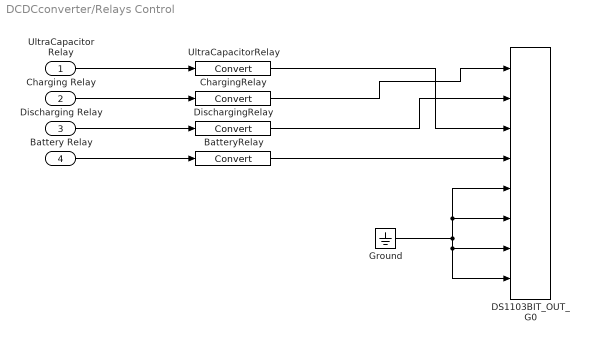
== system DCDCconverter/Relays Control ==
  UltraCapacitor Relay : Inport
  Charging Relay : Inport  Port=2
  Discharging Relay : Inport  Port=3
  Battery Relay : Inport  Port=4
  BatteryRelay : DataTypeConversion
  ChargingRelay : DataTypeConversion
  DS1103BIT_OUT_G0 : rtilib1103/DS1103 MASTER PPC/DS1103BIT_OUT_G0  GroupNo=0  InitValue=[0 0 0 0 0 0 0 0]  TermMode=[1 1 1 1 1 1 1 1]  TermValue=[0 0 0 0 0 0 0 0]  Reserved1=[]  Reserved2=[]  Reserved3=[]  Reserved=[]  DialogFcn=gui1103bit_out  UnitName={ 'DS1103BIT_OUT_G'}  UnitValues={ 0 }  DSProperties=struct('RTI',struct('Version',uint32(1),'BlockType',struct('isSLSource',uint8(0),'isSLSink',uint8(1),'isHWSource',uint8(0),'isHWSink',uint8(1),'isSetup',uint8(0),'isInline',uint8(1),'isNonInline',uint8(0),'isInterrupt',uint8(0),'isChannelwise',uint8(0)),'IOBoardType','DS1103MASTER','UnitType','BIT','Identifier','BITOUT','DialogType','ML','BlockSet','NONE','SlaveProcessor','NONE'))
  DischargingRelay : DataTypeConversion
  Ground : Ground
  UltraCapacitorRelay : DataTypeConversion
  wires:
  Ground/1 -> DS1103BIT_OUT_G0/5, DS1103BIT_OUT_G0/6, DS1103BIT_OUT_G0/8, DS1103BIT_OUT_G0/7
  Charging Relay/1 -> ChargingRelay/1
  Battery Relay/1 -> BatteryRelay/1
  UltraCapacitor Relay/1 -> UltraCapacitorRelay/1
  UltraCapacitorRelay/1 -> DS1103BIT_OUT_G0/3
  Discharging Relay/1 -> DischargingRelay/1
  DischargingRelay/1 -> DS1103BIT_OUT_G0/2
  ChargingRelay/1 -> DS1103BIT_OUT_G0/1
  BatteryRelay/1 -> DS1103BIT_OUT_G0/4

== system DCDCconverter/Subsystem ==
  Vrail : Inport
  Async Rate Transition19 : xpclib/Asynchronous Event/Async Rate Transition  sample_time=Ts2
  Discrete Transfer Fcn1 : DiscreteTransferFcn  Numerator=[1 -1]  Denominator=[Ts2 0]  SampleTime=Ts2
  Discrete Transfer Fcn2 : DiscreteTransferFcn  Numerator=[1 1 1 1 1 1 1 1]  Denominator=[8 0 0 0 0 0 0 0]  SampleTime=Ts2
  Discrete Transfer Fcn3 : DiscreteTransferFcn  Numerator=[1 1 1 1 1 1 1 1]  Denominator=[8 0 0 0 0 0 0 0]  SampleTime=Ts2
  Vrail_filtered : Outport
  dVrail_dT_filtered : Outport  Port=2
  wires:
  Discrete Transfer Fcn3/1 -> Vrail_filtered/1
  Vrail/1 -> Async Rate Transition19/1
  Discrete Transfer Fcn1/1 -> Discrete Transfer Fcn2/1
  Discrete Transfer Fcn2/1 -> dVrail_dT_filtered/1
  Async Rate Transition19/1 -> Discrete Transfer Fcn1/1, Discrete Transfer Fcn3/1

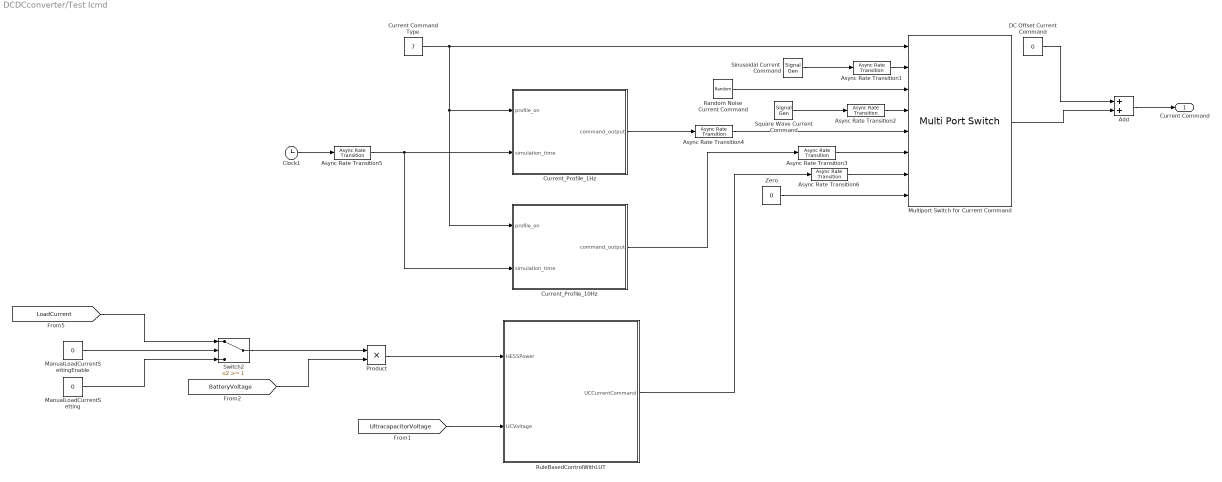
== system DCDCconverter/Test Icmd ==
  Add : Sum
  Async Rate Transition{1..6} (6 alike) : xpclib/Asynchronous Event/Async Rate Transition  sample_time=Ts
  Clock1 : Clock
  Current Command Type : Constant  Value=7  SampleTime=Ts
  Current_Profile_10Hz : MATLAB Function  TreatAsAtomicUnit=on  SystemSampleTime=Ts
  Current_Profile_1Hz : MATLAB Function  TreatAsAtomicUnit=on  SystemSampleTime=Ts
  DC Offset Current Command : Constant  Value=0  SampleTime=Ts
  ManualLoadCurrentSetting : Constant  Value=0  SampleTime=-1
  ManualLoadCurrentSettingEnable : Constant  Value=0  SampleTime=-1
  Multiport Switch for Current Command : MultiPortSwitch  Inputs=7
  Product : Product  RndMeth=Zero
  Random Noise Current Command : UniformRandomNumber  Minimum=0  SampleTime=Ts
  RuleBasedControlWithLUT : Subsystem
  Sinusoidal Current Command : SignalGenerator  Amplitude=0
  Square Wave Current Command : SignalGenerator  WaveForm=square  Amplitude=0
  Switch2 : Switch  Threshold=1  OutDataTypeStr=Inherit: Inherit via back propagation
  Zero : Constant  Value=0  SampleTime=Ts
  Current Command : Outport
  wires:
  Add/1 -> Current Command/1
  Multiport Switch for Current Command/1 -> Add/2
  DC Offset Current Command/1 -> Add/1
  Current Command Type/1 -> Current_Profile_10Hz/1(profile_on), Current_Profile_1Hz/1(profile_on), Multiport Switch for Current Command/1
  Square Wave Current Command/1 -> Async Rate Transition2/1
  Sinusoidal Current Command/1 -> Async Rate Transition1/1
  Random Noise Current Command/1 -> Multiport Switch for Current Command/3
  Async Rate Transition2/1 -> Multiport Switch for Current Command/4
  Async Rate Transition1/1 -> Multiport Switch for Current Command/2
  Current_Profile_1Hz/1(command_output) -> Async Rate Transition4/1
  Current_Profile_10Hz/1(command_output) -> Async Rate Transition3/1
  Async Rate Transition3/1 -> Multiport Switch for Current Command/6
  Async Rate Transition4/1 -> Multiport Switch for Current Command/5
  Clock1/1 -> Async Rate Transition5/1
  Async Rate Transition5/1 -> Current_Profile_1Hz/2(simulation_time), Current_Profile_10Hz/2(simulation_time)
  Zero/1 -> Multiport Switch for Current Command/8
  Async Rate Transition6/1 -> Multiport Switch for Current Command/7
  RuleBasedControlWithLUT/1(UCCurrentCommand) -> Async Rate Transition6/1
  [UltracapacitorVoltage] -> RuleBasedControlWithLUT/2(UCVoltage)
  [BatteryVoltage] -> Product/2
  Product/1 -> RuleBasedControlWithLUT/1(HESSPower)
  Switch2/1 -> Product/1
  [LoadCurrent] -> Switch2/1
  ManualLoadCurrentSettingEnable/1 -> Switch2/2
  ManualLoadCurrentSetting/1 -> Switch2/3

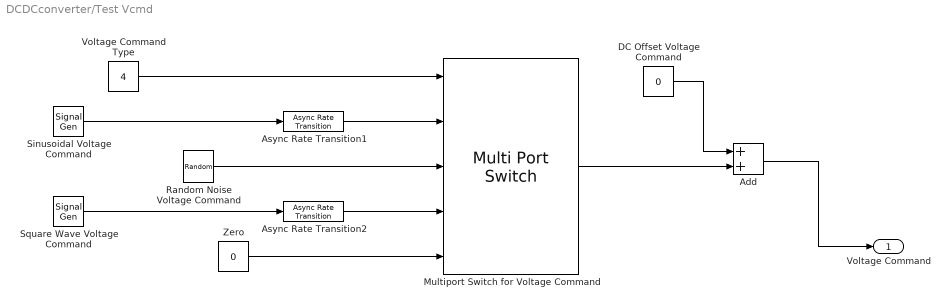
== system DCDCconverter/Test Vcmd ==
  Add : Sum  SampleTime=Ts2
  Async Rate Transition1 : xpclib/Asynchronous Event/Async Rate Transition  sample_time=Ts2
  Async Rate Transition2 : xpclib/Asynchronous Event/Async Rate Transition  sample_time=Ts2
  DC Offset Voltage Command : Constant  Value=0  SampleTime=Ts2
  Multiport Switch for Voltage Command : MultiPortSwitch  Inputs=4  SampleTime=Ts2
  Random Noise Voltage Command : UniformRandomNumber  Minimum=0  SampleTime=Ts2
  Sinusoidal Voltage Command : SignalGenerator  Amplitude=0
  Square Wave Voltage Command : SignalGenerator  WaveForm=square  Amplitude=0
  Voltage Command Type : Constant  Value=4
  Zero : Constant  Value=0
  Voltage Command : Outport
  wires:
  Voltage Command Type/1 -> Multiport Switch for Voltage Command/1
  DC Offset Voltage Command/1 -> Add/1
  Multiport Switch for Voltage Command/1 -> Add/2
  Add/1 -> Voltage Command/1
  Square Wave Voltage Command/1 -> Async Rate Transition2/1
  Sinusoidal Voltage Command/1 -> Async Rate Transition1/1
  Random Noise Voltage Command/1 -> Multiport Switch for Voltage Command/3
  Async Rate Transition2/1 -> Multiport Switch for Voltage Command/4
  Zero/1 -> Multiport Switch for Voltage Command/5
  Async Rate Transition1/1 -> Multiport Switch for Voltage Command/2

== system DCDCconverter/Circuit Outputs/Battery_Current ==
  ZeroCmd : Inport
  Add : Sum  Inputs=-+
  "C18 " : rtilib1103/DS1103 MASTER PPC/DS1103ADC_C17  ChannelNo=18  TimerAPreTrigger=0  Reserved2=[]  Reserved3=[]  Reserved4=[]  DialogFcn=gui1103adc  UnitName={ 'DS1103ADC_C' }  UnitValues={ 18 }  DSProperties=struct('RTI',struct('Version',uint32(1),'BlockType',struct('isSLSource',uint8(1),'isSLSink',uint8(0),'isHWSource',uint8(1),'isHWSink',uint8(0),'isSetup',uint8(0),'isInline',uint8(1),'isNonInline',uint8(0),'isInterrupt',uint8(0),'isChannelwise',uint8(1)),'IOBoardType','DS1103MASTER','UnitType','ADC','Identifier','ADC','DialogType','ML','BlockSet','NONE','SlaveProcessor','NONE'))
  Current Sensor Scaling : Gain  Gain=318.4713
  Data Store Memory : DataStoreMemory  DataStoreName=Offset  ReadBeforeWriteMsg=warning  WriteAfterWriteMsg=warning  WriteAfterReadMsg=warning  DataLoggingName=Data
      settings: DataLoggingMaxPoints=10
  Data Store Read : DataStoreRead  DataStoreName=Offset
  Lowpass Filter : Subsystem  DialogController=fdesignblkfcn  InitFcn=fdesignblkfcn(gcbh, {'InitFcn'});  mask(Lowpass Filter){}
      mask help: Design a lowpass filter
      settings: CopyFcn=fdesignblkfcn(gcbh, {'CopyFcn'});
      mask Help: helpview(mapfilelocation('dsp'), 'dsplowpassfilter');
      mask Display: disp('Lowpass')
  Sample and Hold : dspsigops/Sample and Hold  trig=Rising edge  initCond=0  latchinput=off
  Zeroing : DataStoreWrite  DataStoreName=Offset
  Battery_Current : Outport
  wires:
  ZeroCmd/1 -> Sample and Hold/Trigger
  Add/1 -> Current Sensor Scaling/1
  Sample and Hold/1 -> Zeroing/1
  Current Sensor Scaling/1 -> Battery_Current/1
  Lowpass Filter/1(Out) -> Add/2, Sample and Hold/1
  Data Store Read/1 -> Add/1
  "C18 "/1 -> Lowpass Filter/1(In)

== system DCDCconverter/Circuit Outputs/Battery_Voltage ==
  ZeroCmd : Inport
  Add : Sum  Inputs=-+
  C19 : rtilib1103/DS1103 MASTER PPC/DS1103ADC_C17  ChannelNo=19  TimerAPreTrigger=0  Reserved2=[]  Reserved3=[]  Reserved4=[]  DialogFcn=gui1103adc  UnitName={ 'DS1103ADC_C' }  UnitValues={ 19 }  DSProperties=struct('RTI',struct('Version',uint32(1),'BlockType',struct('isSLSource',uint8(1),'isSLSink',uint8(0),'isHWSource',uint8(1),'isHWSink',uint8(0),'isSetup',uint8(0),'isInline',uint8(1),'isNonInline',uint8(0),'isInterrupt',uint8(0),'isChannelwise',uint8(1)),'IOBoardType','DS1103MASTER','UnitType','ADC','Identifier','ADC','DialogType','ML','BlockSet','NONE','SlaveProcessor','NONE'))
  Data Store Memory : DataStoreMemory  DataStoreName=Offset  ReadBeforeWriteMsg=warning  WriteAfterWriteMsg=warning  WriteAfterReadMsg=warning  DataLoggingName=Data
      settings: DataLoggingMaxPoints=10
  Data Store Read : DataStoreRead  DataStoreName=Offset
  Lowpass Filter : Subsystem  DialogController=fdesignblkfcn  InitFcn=fdesignblkfcn(gcbh, {'InitFcn'});  mask(Lowpass Filter){}
      mask help: Design a lowpass filter
      settings: CopyFcn=fdesignblkfcn(gcbh, {'CopyFcn'});
      mask Help: helpview(mapfilelocation('dsp'), 'dsplowpassfilter');
      mask Display: disp('Lowpass')
  Sample and Hold : dspsigops/Sample and Hold  trig=Rising edge  initCond=0  latchinput=off
  Voltage Sensor Scaling : Gain  Gain=859.9068
  Zeroing : DataStoreWrite  DataStoreName=Offset
  Battery_Voltage : Outport
  wires:
  ZeroCmd/1 -> Sample and Hold/Trigger
  Add/1 -> Voltage Sensor Scaling/1
  Sample and Hold/1 -> Zeroing/1
  Lowpass Filter/1(Out) -> Add/2, Sample and Hold/1
  C19/1 -> Lowpass Filter/1(In)
  Data Store Read/1 -> Add/1
  Voltage Sensor Scaling/1 -> Battery_Voltage/1

== system DCDCconverter/Circuit Outputs/Load_Current ==
  ZeroCmd : Inport
  Add : Sum  Inputs=-+
  C13 : rtilib1103/DS1103 MASTER PPC/DS1103MUX_ADC_CON1  ConverterNo=4  ChannelNos=1  TimerAPreTrigger=0  Reserved2=[]  Reserved3=[]  Reserved4=[]  DialogFcn=gui1103mux_adc  UnitName={ 'DS1103MUX_ADC_CON' }  UnitValues={ 4 }  DSProperties=struct('RTI',struct('Version',uint32(1),'BlockType',struct('isSLSource',uint8(1),'isSLSink',uint8(0),'isHWSource',uint8(1),'isHWSink',uint8(0),'isSetup',uint8(0),'isInline',uint8(1),'isNonInline',uint8(0),'isInterrupt',uint8(0),'isChannelwise',uint8(0)),'IOBoardType','DS1103MASTER','UnitType','ADC','Identifier','ADCMUX','DialogType','ML','BlockSet','NONE','SlaveProcessor','NONE'))
  Current Sensor Scaling : Gain  Gain=796.1782
  Data Store Memory : DataStoreMemory  DataStoreName=Offset  ReadBeforeWriteMsg=warning  WriteAfterWriteMsg=warning  WriteAfterReadMsg=warning  DataLoggingName=Data
      settings: DataLoggingMaxPoints=10
  Data Store Read : DataStoreRead  DataStoreName=Offset
  Lowpass Filter : Subsystem  DialogController=fdesignblkfcn  InitFcn=fdesignblkfcn(gcbh, {'InitFcn'});  mask(Lowpass Filter){}
      mask help: Design a lowpass filter
      settings: CopyFcn=fdesignblkfcn(gcbh, {'CopyFcn'});
      mask Help: helpview(mapfilelocation('dsp'), 'dsplowpassfilter');
      mask Display: disp('Lowpass')
  Sample and Hold : dspsigops/Sample and Hold  trig=Rising edge  initCond=0  latchinput=off
  Zeroing : DataStoreWrite  DataStoreName=Offset
  Load_Current : Outport
  wires:
  Current Sensor Scaling/1 -> Load_Current/1
  C13/1 -> Lowpass Filter/1(In)
  Data Store Read/1 -> Add/1
  Lowpass Filter/1(Out) -> Sample and Hold/1, Add/2
  Sample and Hold/1 -> Zeroing/1
  Add/1 -> Current Sensor Scaling/1
  ZeroCmd/1 -> Sample and Hold/Trigger

== system DCDCconverter/Circuit Outputs/UltraCapacitor_Current ==
  ZeroCmd : Inport
  Add : Sum  Inputs=-+
  C17 : rtilib1103/DS1103 MASTER PPC/DS1103ADC_C17  ChannelNo=17  TimerAPreTrigger=0  Reserved2=[]  Reserved3=[]  Reserved4=[]  DialogFcn=gui1103adc  UnitName={ 'DS1103ADC_C' }  UnitValues={ 17 }  DSProperties=struct('RTI',struct('Version',uint32(1),'BlockType',struct('isSLSource',uint8(1),'isSLSink',uint8(0),'isHWSource',uint8(1),'isHWSink',uint8(0),'isSetup',uint8(0),'isInline',uint8(1),'isNonInline',uint8(0),'isInterrupt',uint8(0),'isChannelwise',uint8(1)),'IOBoardType','DS1103MASTER','UnitType','ADC','Identifier','ADC','DialogType','ML','BlockSet','NONE','SlaveProcessor','NONE'))
  Current Sensor Scaling : Gain  Gain=318.4713
  Data Store Memory : DataStoreMemory  DataStoreName=Offset  ReadBeforeWriteMsg=warning  WriteAfterWriteMsg=warning  WriteAfterReadMsg=warning  DataLoggingName=Data
      settings: DataLoggingMaxPoints=10
  Data Store Read : DataStoreRead  DataStoreName=Offset
  Lowpass Filter : Subsystem  DialogController=fdesignblkfcn  InitFcn=fdesignblkfcn(gcbh, {'InitFcn'});  mask(Lowpass Filter){}
      mask help: Design a lowpass filter
      settings: CopyFcn=fdesignblkfcn(gcbh, {'CopyFcn'});
      mask Help: helpview(mapfilelocation('dsp'), 'dsplowpassfilter');
      mask Display: disp('Lowpass')
  Sample and Hold : dspsigops/Sample and Hold  trig=Rising edge  initCond=0  latchinput=off
  Zeroing : DataStoreWrite  DataStoreName=Offset
  Ultracapacitor_Current : Outport
  wires:
  ZeroCmd/1 -> Sample and Hold/Trigger
  Add/1 -> Current Sensor Scaling/1
  Sample and Hold/1 -> Zeroing/1
  Lowpass Filter/1(Out) -> Add/2, Sample and Hold/1
  Data Store Read/1 -> Add/1
  C17/1 -> Lowpass Filter/1(In)
  Current Sensor Scaling/1 -> Ultracapacitor_Current/1

== system DCDCconverter/Circuit Outputs/UltraCapacitor_Voltage ==
  ZeroCmd : Inport
  Add : Sum  Inputs=-+
  C20 : rtilib1103/DS1103 MASTER PPC/DS1103ADC_C17  ChannelNo=20  TimerAPreTrigger=0  Reserved2=[]  Reserved3=[]  Reserved4=[]  DialogFcn=gui1103adc  UnitName={ 'DS1103ADC_C' }  UnitValues={ 20 }  DSProperties=struct('RTI',struct('Version',uint32(1),'BlockType',struct('isSLSource',uint8(1),'isSLSink',uint8(0),'isHWSource',uint8(1),'isHWSink',uint8(0),'isSetup',uint8(0),'isInline',uint8(1),'isNonInline',uint8(0),'isInterrupt',uint8(0),'isChannelwise',uint8(1)),'IOBoardType','DS1103MASTER','UnitType','ADC','Identifier','ADC','DialogType','ML','BlockSet','NONE','SlaveProcessor','NONE'))
  Data Store Memory : DataStoreMemory  DataStoreName=Offset  ReadBeforeWriteMsg=warning  WriteAfterWriteMsg=warning  WriteAfterReadMsg=warning  DataLoggingName=Data
      settings: DataLoggingMaxPoints=10
  Data Store Read : DataStoreRead  DataStoreName=Offset
  Lowpass Filter : Subsystem  DialogController=fdesignblkfcn  InitFcn=fdesignblkfcn(gcbh, {'InitFcn'});  mask(Lowpass Filter){}
      mask help: Design a lowpass filter
      settings: CopyFcn=fdesignblkfcn(gcbh, {'CopyFcn'});
      mask Help: helpview(mapfilelocation('dsp'), 'dsplowpassfilter');
      mask Display: disp('Lowpass')
  Sample and Hold : dspsigops/Sample and Hold  trig=Rising edge  initCond=0  latchinput=off
  Voltage Sensor Scaling : Gain  Gain=-859.9068
  Zeroing : DataStoreWrite  DataStoreName=Offset
  Ultracapacitor_Voltage : Outport
  wires:
  Lowpass Filter/1(Out) -> Add/2, Sample and Hold/1
  Sample and Hold/1 -> Zeroing/1
  Add/1 -> Voltage Sensor Scaling/1
  ZeroCmd/1 -> Sample and Hold/Trigger
  C20/1 -> Lowpass Filter/1(In)
  Data Store Read/1 -> Add/1
  Voltage Sensor Scaling/1 -> Ultracapacitor_Voltage/1

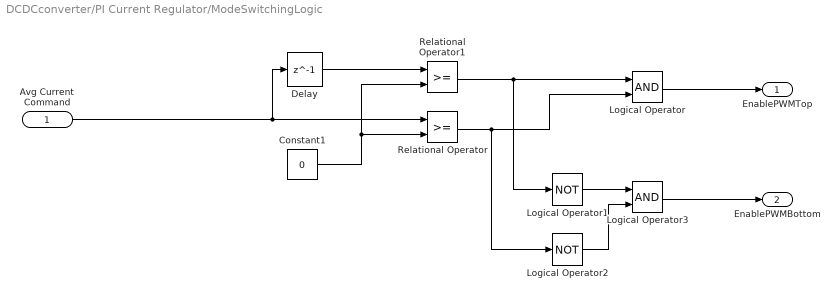
== system DCDCconverter/PI Current Regulator/ModeSwitchingLogic ==
  Avg Current Command : Inport
  Constant1 : Constant  Value=0  SampleTime=Ts
  Delay : Delay  DelayLength=1  SampleTime=Ts
  Logical Operator : Logic  AllPortsSameDT=off  OutDataTypeStr=boolean
  Logical Operator1 : Logic  Operator=NOT  AllPortsSameDT=off  OutDataTypeStr=boolean
  Logical Operator2 : Logic  Operator=NOT  AllPortsSameDT=off  OutDataTypeStr=boolean
  Logical Operator3 : Logic  AllPortsSameDT=off  OutDataTypeStr=boolean
  Relational Operator : RelationalOperator  OutDataTypeStr=boolean
  Relational Operator1 : RelationalOperator  OutDataTypeStr=boolean
  EnablePWMTop : Outport
  EnablePWMBottom : Outport  Port=2
  wires:
  Relational Operator1/1 -> Logical Operator1/1, Logical Operator/1
  Constant1/1 -> Relational Operator/2, Relational Operator1/2
  Logical Operator2/1 -> Logical Operator3/2
  Logical Operator1/1 -> Logical Operator3/1
  Avg Current Command/1 -> Delay/1, Relational Operator/1
  Relational Operator/1 -> Logical Operator2/1, Logical Operator/2
  Delay/1 -> Relational Operator1/1
  Logical Operator/1 -> EnablePWMTop/1
  Logical Operator3/1 -> EnablePWMBottom/1

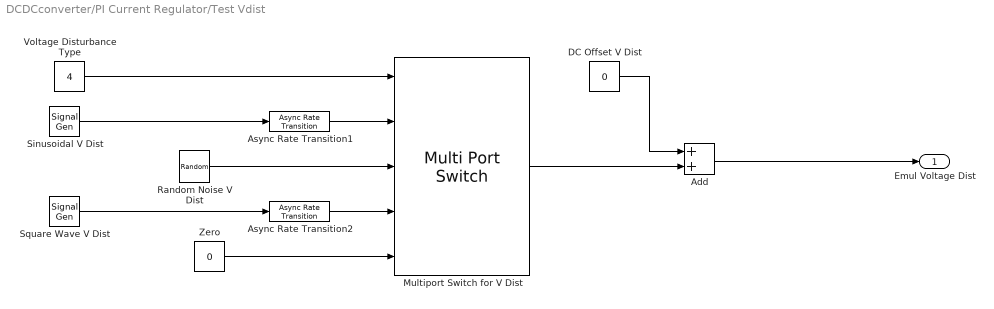
== system DCDCconverter/PI Current Regulator/Test Vdist ==
  Add : Sum
  Async Rate Transition1 : xpclib/Asynchronous Event/Async Rate Transition  sample_time=Ts
  Async Rate Transition2 : xpclib/Asynchronous Event/Async Rate Transition  sample_time=Ts
  DC Offset V Dist : Constant  Value=0  SampleTime=Ts
  Multiport Switch for V Dist : MultiPortSwitch  Inputs=4  SampleTime=Ts
  Random Noise V Dist : UniformRandomNumber  Minimum=0  SampleTime=Ts
  Sinusoidal V Dist : SignalGenerator  Amplitude=0
  Square Wave V Dist : SignalGenerator  WaveForm=square  Amplitude=0
  Voltage Disturbance Type : Constant  Value=4  SampleTime=Ts
  Zero : Constant  Value=0  SampleTime=Ts
  Emul Voltage Dist : Outport
  wires:
  Add/1 -> Emul Voltage Dist/1
  Multiport Switch for V Dist/1 -> Add/2
  DC Offset V Dist/1 -> Add/1
  Voltage Disturbance Type/1 -> Multiport Switch for V Dist/1
  Square Wave V Dist/1 -> Async Rate Transition2/1
  Sinusoidal V Dist/1 -> Async Rate Transition1/1
  Random Noise V Dist/1 -> Multiport Switch for V Dist/3
  Async Rate Transition2/1 -> Multiport Switch for V Dist/4
  Zero/1 -> Multiport Switch for V Dist/5
  Async Rate Transition1/1 -> Multiport Switch for V Dist/2

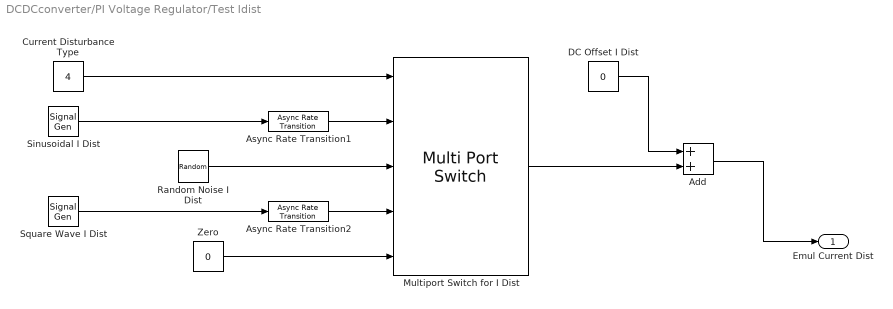
== system DCDCconverter/PI Voltage Regulator/Test Idist ==
  Add : Sum
  Async Rate Transition1 : xpclib/Asynchronous Event/Async Rate Transition  sample_time=Ts2
  Async Rate Transition2 : xpclib/Asynchronous Event/Async Rate Transition  sample_time=Ts2
  Current Disturbance Type : Constant  Value=4  SampleTime=Ts2
  DC Offset I Dist : Constant  Value=0  SampleTime=Ts2
  Multiport Switch for I Dist : MultiPortSwitch  Inputs=4  SampleTime=Ts2
  Random Noise I Dist : UniformRandomNumber  Minimum=0  SampleTime=Ts2
  Sinusoidal I Dist : SignalGenerator  Amplitude=0
  Square Wave I Dist : SignalGenerator  WaveForm=square  Amplitude=0
  Zero : Constant  Value=0  SampleTime=Ts2
  Emul Current Dist : Outport
  wires:
  Add/1 -> Emul Current Dist/1
  Multiport Switch for I Dist/1 -> Add/2
  DC Offset I Dist/1 -> Add/1
  Current Disturbance Type/1 -> Multiport Switch for I Dist/1
  Square Wave I Dist/1 -> Async Rate Transition2/1
  Sinusoidal I Dist/1 -> Async Rate Transition1/1
  Random Noise I Dist/1 -> Multiport Switch for I Dist/3
  Async Rate Transition2/1 -> Multiport Switch for I Dist/4
  Zero/1 -> Multiport Switch for I Dist/5
  Async Rate Transition1/1 -> Multiport Switch for I Dist/2
